simulink model "simulink_differintial_controller"  (R2018a)
settings: Solver=ode45  StartTime=0.0  StopTime=50  FixedStep=.01  MaxStep=.01  RelTol=1e-3
values from neighbouring files (symbols this model uses):
  initparam = [pi/2;.5;0]    [init.m]
libraries: simulink x2
settings Model: Creator=yadav  LastModifiedBy=e.amutete
settings OptimizationCC: LifeSpan=inf
settings DebuggingCC: SFExecutionAtInitializationDiag=none
settings CodeAppCC: StateflowObjectComments=on

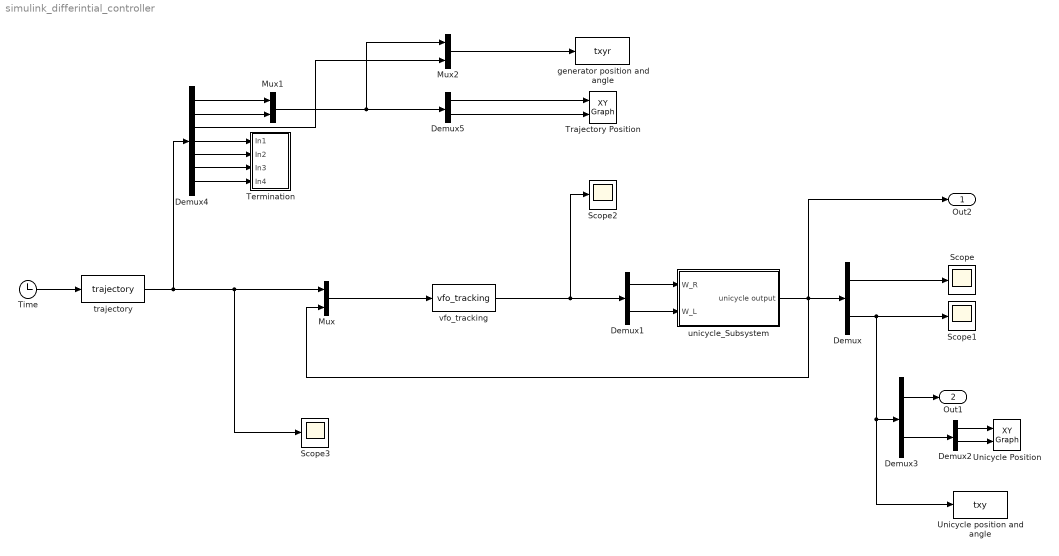
== system simulink_differintial_controller ==
  Demux{,1..2,5} (4 alike) : Demux  Outputs=2
  Demux3 : Demux  Outputs=[1;2]
  Demux4 : Demux  Outputs=7
  Mux : Mux  Inputs=2
  Mux1 : Mux  Inputs=2
  Mux2 : Mux  Inputs=2
  Scope{,1..3} (4 alike) : Scope
  Termination : Subsystem
  Time : Clock
  Trajectory Position : simulink/Sinks/XY Graph  xmin=-5  xmax=5  ymin=-5  ymax=5  st=-1
  Unicycle Position : simulink/Sinks/XY Graph  xmin=-5  xmax=5  ymin=-5  ymax=5  st=-1
  Unicycle position and angle : ToWorkspace  VariableName=txy  SaveFormat=Timeseries  SampleTime=-1
  generator position and angle : ToWorkspace  VariableName=txyr  SaveFormat=Timeseries  SampleTime=-1
  "trajectory " : MATLABFcn  MATLABFcn=trajectory
  unicycle_Subsystem : Subsystem
  vfo_tracking : MATLABFcn  MATLABFcn=vfo_tracking
  Out2 : Outport
  Out1 : Outport  Port=2
  wires:
  Demux/2 -> Unicycle position and angle/1, Demux3/1, Scope1/1
  Demux/1 -> Scope/1
  Demux1/2 -> unicycle_Subsystem/2(W_L)
  Demux1/1 -> unicycle_Subsystem/1(W_R)
  unicycle_Subsystem/1(unicycle output) -> Demux/1, Out2/1, Mux/2
  Time/1 -> "trajectory "/1
  "trajectory "/1 -> Scope3/1, Mux/1, Demux4/1
  Demux2/1 -> Unicycle Position/1
  Demux2/2 -> Unicycle Position/2
  Demux3/2 -> Demux2/1
  Demux3/1 -> Out1/1
  Demux4/1 -> Mux1/1
  Demux4/2 -> Mux1/2
  Mux1/1 -> Mux2/1, Demux5/1
  Demux5/1 -> Trajectory Position/1
  Mux2/1 -> generator position and angle/1
  Demux4/4 -> Termination/1(In1)
  Demux4/5 -> Termination/2(In2)
  Demux4/6 -> Termination/3(In3)
  Demux4/7 -> Termination/4(In4)
  Demux5/2 -> Trajectory Position/2
  Demux4/3 -> Mux2/2
  vfo_tracking/1 -> Scope2/1, Demux1/1
  Mux/1 -> vfo_tracking/1

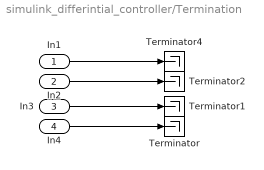
== system simulink_differintial_controller/Termination ==
  In1 : Inport
  In2 : Inport  Port=2
  In3 : Inport  Port=3
  In4 : Inport  Port=4
  Terminator{,1..2,4} (4 alike) : Terminator
  wires:
  In4/1 -> Terminator/1
  In3/1 -> Terminator1/1
  In1/1 -> Terminator4/1
  In2/1 -> Terminator2/1

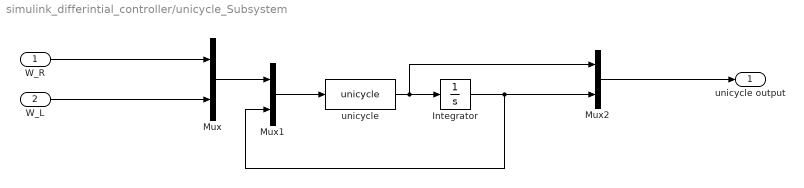
== system simulink_differintial_controller/unicycle_Subsystem ==
  W_R : Inport
  W_L : Inport  Port=2
  Integrator : Integrator  InitialCondition=initparam
  Mux : Mux  Inputs=2
  Mux1 : Mux  Inputs=2
  Mux2 : Mux  Inputs=2
  "unicycle " : MATLABFcn  MATLABFcn=unicycle
  unicycle output : Outport
  wires:
  W_L/1 -> Mux/2
  "unicycle "/1 -> Integrator/1, Mux2/1
  Mux/1 -> Mux1/1
  Integrator/1 -> Mux2/2, Mux1/2
  Mux1/1 -> "unicycle "/1
  W_R/1 -> Mux/1
  Mux2/1 -> unicycle output/1
